simulink model "test_model"  (R2022b)
settings: Solver=ode5  StartTime=0.0  StopTime=5  RelTol=1e-3
settings Model: SimulationMode=external  Creator=ehandyca  LastModifiedBy=ehandyca
settings HardwareCC: ProdBitPerLong=64  ProdHWDeviceType=Intel->x86-64 (Linux 64)
settings RTWCC: Description=Simulink Desktop Real-Time  SystemTargetFile=sldrt.tlc  TemplateMakefile=sldrt.tmf  RTWCompilerOptimization=on
settings CodeAppCC: MaxIdLength=95
settings SimulinkDesktopRealTimeCC: TargetLibSuffix=_sldrt.a  TargetPreCompLibLocation=C:\Program Files\MATLAB\R2022b\toolbox\sldrt\lib\win64

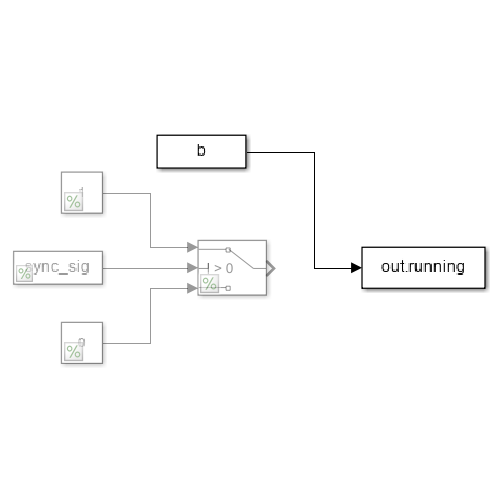
[thumbnail: Simulink's stored preview of the top-level diagram]
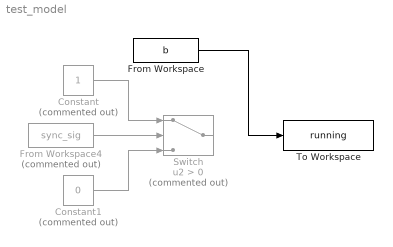
== system test_model ==
  Constant : Constant  Commented=on
  Constant1 : Constant  Commented=on  Value=0
  From Workspace : FromWorkspace  VariableName=b
  From Workspace4 : FromWorkspace  Commented=on  VariableName=sync_sig
  Switch : Switch  Commented=on  Criteria=u2 > Threshold  SaturateOnIntegerOverflow=off  InputSameDT=off
  To Workspace : ToWorkspace  VariableName=running  SampleTime=-1
  wires:
  From Workspace4/1 -> Switch/2
  Constant1/1 -> Switch/3
  Constant/1 -> Switch/1
  From Workspace/1 -> To Workspace/1
